simulink model "simple_pll_3"  (Simulink 7.4)
settings: Solver=ode45  StartTime=0.0  StopTime=5e-6  MaxStep=1/(10*800e6)  RelTol=.001
PreLoadFcn:
  |  [a,b]=ellip(5,1,60,2*pi*40e6,'s');
StartFcn:
  | tic;
StopFcn:
  | pll_sim_time=toc
undefined symbols (not defined in the file or in its folder): a, b, Fs, sided, Two
libraries: powerlib x10, simulink x3, simulink_extras x2, dsparch4 x2, dspsnks4 x1, commsynccomp2 x1
settings Model: Creator=dbenson  LastModifiedBy=Dick  BufferReuse=off
settings DataIOCC: LimitDataPoints=off  SaveOutput=off  SaveTime=off  OutputSaveName=vco_control  SignalLoggingName=sigsOut
settings OptimizationCC: BooleanDataType=off  OptimizeBlockIOStorage=off  BufferReuse=off  EnforceIntegerDowncast=off  ExpressionFolding=off  FoldNonRolledExpr=off  LocalBlockOutputs=off  InitFltsAndDblsToZero=on
settings DebuggingCC: SaveWithParameterizedLinksMsg=none  SignalResolutionControl=TryResolveAllWithWarning  SolverPrmCheckMsg=none  MultiTaskDSMMsg=warning  MultiTaskCondExecSysMsg=none  StrictBusMsg=None
settings HardwareCC: TargetUnknown=on
settings RTWCC: IncludeERTFirstTime=on
settings GRTTargetCC: TargetFcnLib=ansi_tfl_tmw.mat

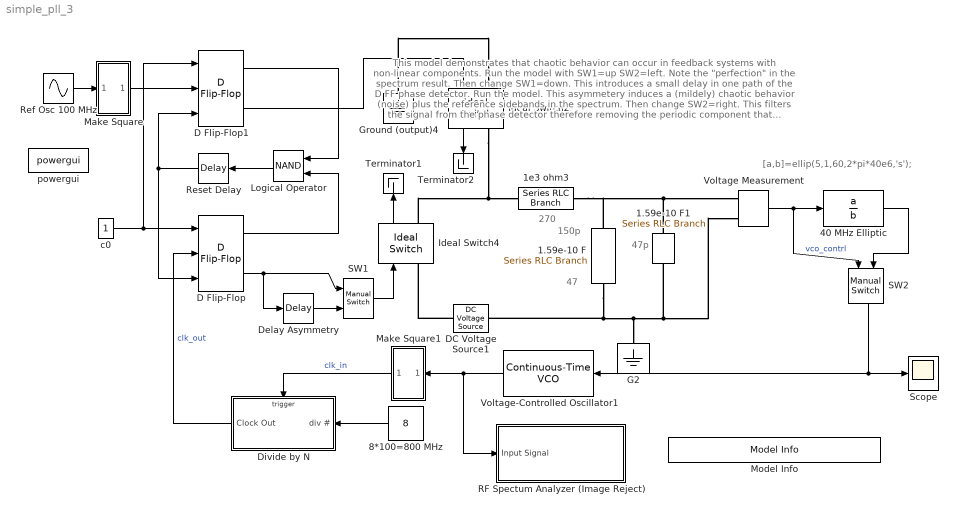
== system simple_pll_3 ==
  note: [a,b]=ellip(5,1,60,2*pi*40e6,'s');
  note: This model demonstrates that chaotic behavior can occur in feedback systems
      | with non-linear components.
      |
      | Run the model with SW1=up SW2=left. Note the "perfection" in the
      | spectrum result.  Then change SW1=down. This introduces a small delay
      | in one path of the D FF phase detector.  Run the model. This asymmetery
      | induces a (mildely) chaotic behavior (noise) plus the reference sidebands
      | in the spectrum.  Then change SW2=right.  This filters the signal from the
      | phase detector therefore removing the periodic component that  produces
      | the sidebands. However the noise due to the chaotic process is still present
      | in the passband of the filter.
  note: 270
  note: 150p
  note: 47
  note: 47p
  1.59e-10 F : powerlib/Elements/Series RLC Branch  DialogController=POWERSYS.PowerSysDialog  PhysicalDomain=powersysdomain  SubClassName=unknown  LeftPortType=p1  RightPortType=p1  LConnTagsString=__new0  RConnTagsString=__new0  BranchType=RC  Resistance=47  Inductance=1.0  SetiL0=off  InitialCurrent=0  Capacitance=150e-12  Setx0=off  InitialVoltage=0  Measurements=None
  1.59e-10 F1 : powerlib/Elements/Series RLC Branch  DialogController=POWERSYS.PowerSysDialog  PhysicalDomain=powersysdomain  SubClassName=unknown  LeftPortType=p1  RightPortType=p1  LConnTagsString=__new0  RConnTagsString=__new0  BranchType=C  Resistance=1.0  Inductance=1.0  SetiL0=off  InitialCurrent=0  Capacitance=47e-12  Setx0=off  InitialVoltage=0  Measurements=None
  1e3 ohm3 : powerlib/Elements/Series RLC Branch  DialogController=POWERSYS.PowerSysDialog  PhysicalDomain=powersysdomain  SubClassName=unknown  LeftPortType=p1  RightPortType=p1  LConnTagsString=__new0  RConnTagsString=__new0  BranchType=R  Resistance=270  Inductance=1.0  SetiL0=off  InitialCurrent=0  Capacitance=1.0  Setx0=off  InitialVoltage=0  Measurements=None
  "40 MHz Elliptic " : TransferFcn  Numerator=a  Denominator=b
  "8*100=800 MHz " : Constant  Value=8  OutDataType=sfix(16)  OutScaling=2^0
  D Flip-Flop : simulink_extras/Flip Flops/D Flip-Flop  SystemSampleTime=-1
  D Flip-Flop1 : simulink_extras/Flip Flops/D Flip-Flop  SystemSampleTime=-1
  DC Voltage Source1 : powerlib/Electrical Sources/DC Voltage Source  Description=source block  DialogController=POWERSYS.PowerSysDialog  SystemSampleTime=-1  Amplitude=5  Measurements=None
      settings: AttributesFormatString=\n
  Delay Asymmetry : TransportDelay  DelayTime=100e-12  BufferSize=100
  Divide by N : Subsystem  AncestorBlock=rab_favorites/Divide by N  TreatAsAtomicUnit=on
  G2 : powerlib/Elements/Ground  DialogController=POWERSYS.PowerSysDialog  PhysicalDomain=powersysdomain  SubClassName=unknown  LeftPortType=p1  RightPortType=p1  LConnTagsString=a
  Ground (output)4 : powerlib/Elements/Ground  DialogController=POWERSYS.PowerSysDialog  PhysicalDomain=powersysdomain  SubClassName=unknown  LeftPortType=p1  RightPortType=p1  LConnTagsString=a
  Ideal Switch2 : powerlib/Power Electronics/Ideal Switch  DialogController=POWERSYS.PowerSysDialog  SystemSampleTime=-1  Ron=180  Lon=1e-007  IC=1  Rs=0  Cs=0  Measurements=on
      settings: AttributesFormatString=\n
  Ideal Switch4 : powerlib/Power Electronics/Ideal Switch  DialogController=POWERSYS.PowerSysDialog  SystemSampleTime=-1  Ron=180  Lon=1e-007  IC=0  Rs=0  Cs=0  Measurements=on
      settings: AttributesFormatString=\n
  Logical Operator : Logic  Operator=NAND
  Make Square : Subsystem
      mask Type: Make Square
      mask Description:
      | For input +ve values output is 1
      | For input -ve values output is 0
      mask Display: plot(0,0,100,100,[90,70,70,50,50,30,30,10,10],[20,20,40,40,20,20,40,40,20],[90,87,84,80,76,73,70,67,63,60,57,53,50,47,44,40,36,33,30,27,23,20,17,13,10],[70,65,63,62,63,65,70,75,77,78,77,75,70,65,63,62,63,65,70,75,77,78,77,75,70])
  Make Square1 : Subsystem
      mask Type: Make Square
      mask Description:
      | For input +ve values output is 1
      | For input -ve values output is 0
      mask Display: plot(0,0,100,100,[90,70,70,50,50,30,30,10,10],[20,20,40,40,20,20,40,40,20],[90,87,84,80,76,73,70,67,63,60,57,53,50,47,44,40,36,33,30,27,23,20,17,13,10],[70,65,63,62,63,65,70,75,77,78,77,75,70,65,63,62,63,65,70,75,77,78,77,75,70])
  Model Info : simulink/Model-Wide Utilities/Model Info  SystemSampleTime=-1  InitialBlockCM=None  BlockCM=None  Frame=on  DisplayStringWithTags=Copywrite 2005-2010 The MathWorks, Inc.  HorizontalTextAlignment=Center  LeftAlignmentValue=0.5  SourceBlockDiagram=simple_pll_3  TagMaxNumber=20
  RF Spectum Analyzer (Image Reject) : Subsystem  Description=Spectrum Analyzer  mask{BW=300e6, Fc=800e6}
      mask prompts: BW "Bandwidth"; Fc "Center Freq"
      mask Display: fprintf('Spectrum Analyzer \n Fc=%7.2f MHz \n BW=%7.2f MHz',Fc/1e6,BW/1e6)
  Ref Osc 100 MHz : Sin  Amplitude=1  Bias=0  Frequency=2*pi*100e6  Phase=pi  Samples=10  SampleTime=0  Offset=0
  "Reset Delay " : TransportDelay  DelayTime=1e-9  InitialOutput=1  BufferSize=100
  SW1 : simulink/Signal Routing/Manual Switch  SystemSampleTime=-1  sw=1  action=0  varsize=off
  "SW2 " : simulink/Signal Routing/Manual Switch  SystemSampleTime=-1  sw=1  action=0  varsize=off
  Scope : Scope
      settings: TimeRange=6e-006  YMin=0  YMax=4  Decimation=100
  Terminator1 : Terminator
  Terminator2 : Terminator
  Voltage Measurement : powerlib/Measurements/Voltage Measurement  Tag=PoWeRsYsTeMmEaSuReMeNt  DialogController=POWERSYS.PowerSysDialog  SystemSampleTime=-1  PhasorSimulation=off  OutputType=Magnitude  PSBequivalent=0
  Voltage-Controlled Oscillator1 : commsynccomp2/Continuous-Time VCO  SystemSampleTime=-1  Ac=1  Fc=8*90e6  Kc=8*20e6/5  Ph=pi
  "c0 " : Constant  OutDataType=sfix(16)  OutScaling=2^0
  powergui : powerlib/powergui  SystemSampleTime=-1  SimulationMode=Continuous  SampleTime=50e-6  frequency=60  SPID=off  DisableSnubberDevices=off  DisableRonSwitches=off  DisableVfSwitches=off  SwTol=0  Interpol=off  frequencyindice=0  echomessages=off  HookPort=off  DisplayEquations=off  FunctionMessages=off  EnableUseOfTLC=off  x0status=blocks  RestoreLinks=warning  Frange=[0:2:500]  Ylog=off  Xlog=on  ShowGrid=off  save=off  variable=ZData  ZoomFFT=on  StartTime=0.0  cycles=1  DisplayStyle=1  fundamental=60  FreqAxis=off  MaxFrequency=1000  frequencyindicesteady=1  RmsSteady=1  display=off  Ts=0  methode=off
  wires:
  Logical Operator/1 -> "Reset Delay "/1
  D Flip-Flop1/1 -> Logical Operator/1
  D Flip-Flop/1 -> Logical Operator/2
  "Reset Delay "/1 -> D Flip-Flop/3, D Flip-Flop1/3
  Make Square/1(Out1) -> D Flip-Flop1/2
  Make Square1/1(Out1) -> Divide by N/Trigger  "clk_in"
  Divide by N/1(Clock Out) -> D Flip-Flop/2  "clk_out"
  "8*100=800 MHz "/1 -> Divide by N/1(div #)
  "c0 "/1 -> D Flip-Flop/1, D Flip-Flop1/1
  D Flip-Flop/2 -> Delay Asymmetry/1, SW1/1
  Ref Osc 100 MHz/1 -> Make Square/1(In1)
  "40 MHz Elliptic "/1 -> "SW2 "/2
  Delay Asymmetry/1 -> SW1/2
  Ideal Switch2/1 -> Terminator2/1
  Ideal Switch4/1 -> Terminator1/1
  D Flip-Flop1/2 -> Ideal Switch2/1
  Voltage Measurement/1 -> "40 MHz Elliptic "/1, "SW2 "/1  "vco_contrl"
  SW1/1 -> Ideal Switch4/1
  Voltage-Controlled Oscillator1/1 -> Make Square1/1(In1), RF Spectum Analyzer (Image Reject)/1(Input Signal)
  "SW2 "/1 -> Voltage-Controlled Oscillator1/1, Scope/1
  connections:
  Ground (output)4/LConn1 -- Ideal Switch2/LConn1
  DC Voltage Source1/RConn1 -- Ideal Switch4/LConn1
  1e3 ohm3/RConn1 -- 1.59e-10 F/RConn1 -- Voltage Measurement/LConn1 -- 1.59e-10 F1/RConn1
  Ideal Switch2/RConn1 -- Ideal Switch4/RConn1 -- 1e3 ohm3/LConn1
  1.59e-10 F/LConn1 -- 1.59e-10 F1/LConn1 -- Voltage Measurement/LConn2 -- G2/LConn1 -- DC Voltage Source1/LConn1

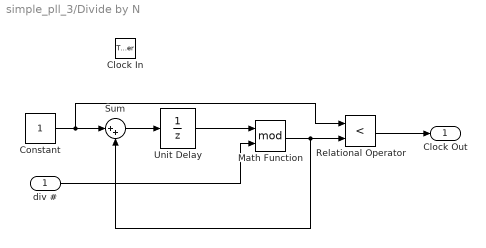
== system simple_pll_3/Divide by N ==
  div # : Inport  OutDataType=sfix(16)  OutScaling=2^0
  Clock In : TriggerPort  TriggerType=falling
  Constant : Constant  OutDataType=sfix(16)  OutScaling=2^0
  Math Function : Math  Operator=mod  OutDataType=sfix(16)  OutScaling=2^0  SaturateOnIntegerOverflow=on
  Relational Operator : RelationalOperator  Operator=<  InputSameDT=on
  Sum : Sum  Inputs=|++  OutDataType=sfix(16)  OutScaling=2^0  SaturateOnIntegerOverflow=on  InputSameDT=on  OutDataTypeStr=Inherit: Same as first input
  Unit Delay : UnitDelay  SampleTime=-1
  Clock Out : Outport  OutDataType=sfix(16)  OutScaling=2^0
  wires:
  Constant/1 -> Sum/1, Relational Operator/1
  Sum/1 -> Unit Delay/1
  Unit Delay/1 -> Math Function/1
  div #/1 -> Math Function/2
  Math Function/1 -> Sum/2, Relational Operator/2
  Relational Operator/1 -> Clock Out/1

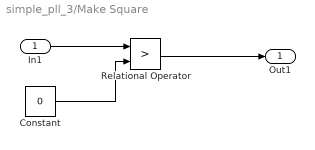
== system simple_pll_3/Make Square ==
  In1 : Inport  OutDataType=sfix(16)  OutScaling=2^0
  Constant : Constant  Value=0  OutDataType=sfix(16)  OutScaling=2^0
  Relational Operator : RelationalOperator  Operator=>  InputSameDT=on
  Out1 : Outport  OutDataType=sfix(16)  OutScaling=2^0
  wires:
  Relational Operator/1 -> Out1/1
  Constant/1 -> Relational Operator/2
  In1/1 -> Relational Operator/1

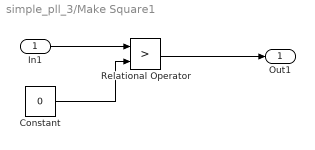
== system simple_pll_3/Make Square1 ==
  In1 : Inport  OutDataType=sfix(16)  OutScaling=2^0
  Constant : Constant  Value=0  OutDataType=sfix(16)  OutScaling=2^0
  Relational Operator : RelationalOperator  Operator=>  InputSameDT=on
  Out1 : Outport  OutDataType=sfix(16)  OutScaling=2^0
  wires:
  In1/1 -> Relational Operator/1
  Constant/1 -> Relational Operator/2
  Relational Operator/1 -> Out1/1

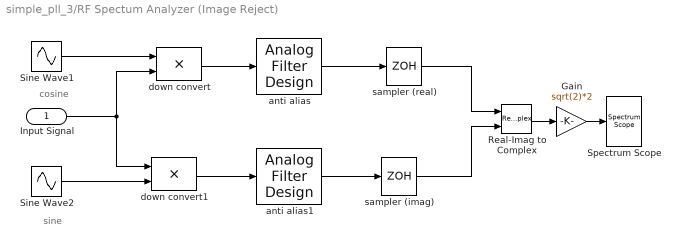
== system simple_pll_3/RF Spectum Analyzer (Image Reject) ==
  note: cosine
  note: sine
  Input Signal : Inport  OutDataType=sfix(16)  OutScaling=2^0
  Gain : Gain  Gain=sqrt(2)*2  ParameterDataType=fixdt(1, 16)  ParameterScaling=2^0  OutDataType=fixdt(1, 16)  OutScaling=2^0
  Real-Imag to Complex : RealImagToComplex
  Sine Wave1 : Sin  Amplitude=1  Bias=0  Frequency=2*pi*(Fc)  Phase=-pi/2  Samples=10  SampleTime=0  Offset=0
  Sine Wave2 : Sin  Amplitude=1  Bias=0  Frequency=2*pi*(Fc)  Phase=0  Samples=10  SampleTime=0  Offset=0
  Spectrum Scope : dspsnks4/Spectrum Scope  DialogController=dspdialog.SpectrumScope  DialogControllerArgs=DataTag0  SystemSampleTime=-1  ScopeProperties=on  Domain=Frequency  HorizSpan=1  UseBuffer=on  BufferSize=256  Overlap=64  inpFftLenInherit=off  FFTlength=128  numAvg=2  DisplayProperties=off  AxisGrid=on  Memory=off  FrameNumber=on  AxisLegend=off  AxisZoom=off  OpenScopeAtSimStart=on  OpenScopeImmediately=off  FigPos=[3 16 504 221]  AxisProperties=off  XUnits=Hertz  XRange=Two-sided ((-Fs/2...Fs/2])  XDisplay=0  InheritXIncr=on  XIncr=1.0  XLabel=Samples  XLimit=Auto  YUnits=dBW  XMax=1  XMin=0  YLabel=dBW  LineProperties=off  wintypeSpecScope=Hann  RsSpecScope=50  betaSpecScope=5  winsampSpecScope=Periodic  XAxisParamsVer=6.8
      settings: YMin=-100  YMax=10
  anti alias : dsparch4/Analog Filter Design  method=Elliptic  filttype=Lowpass  N=9  Wlo=BW*pi  Whi=80  Rp=1.2  Rs=100
  anti alias1 : dsparch4/Analog Filter Design  method=Elliptic  filttype=Lowpass  N=9  Wlo=BW*pi  Whi=80  Rp=1.2  Rs=100
  down convert : Product  OutDataType=sfix(16)  OutScaling=2^0  SaturateOnIntegerOverflow=on  InputSameDT=on  OutDataTypeStr=Inherit: Same as first input
  down convert1 : Product  OutDataType=sfix(16)  OutScaling=2^0  SaturateOnIntegerOverflow=on  InputSameDT=on  OutDataTypeStr=Inherit: Same as first input
  sampler (imag) : ZeroOrderHold  SampleTime=1/(1.28*BW)
  sampler (real) : ZeroOrderHold  SampleTime=1/(1.28*BW)
  wires:
  Input Signal/1 -> down convert/2, down convert1/1
  down convert/1 -> anti alias/1
  anti alias/1 -> sampler (real)/1
  Sine Wave1/1 -> down convert/1
  Sine Wave2/1 -> down convert1/2
  anti alias1/1 -> sampler (imag)/1
  down convert1/1 -> anti alias1/1
  sampler (real)/1 -> Real-Imag to Complex/1
  sampler (imag)/1 -> Real-Imag to Complex/2
  Real-Imag to Complex/1 -> Gain/1
  Gain/1 -> Spectrum Scope/1
